simulink model "vehicleDynamicsModelTest"  (R2019b)
settings: Solver=FixedStepDiscrete  StartTime=0.0  StopTime=15  FixedStep=0.1  RelTol=1e-3
undefined symbols (not defined in the file or in its folder): DiscIntNeverNeededParam, sigbuilder_block
libraries: simulink x2
settings Model: Creator=jasprit  LastModifiedBy=jasprit
settings DataIOCC: ReturnWorkspaceOutputs=off
settings DebuggingCC: ArithmeticOperatorsInVariantConditions=warning
settings SFSimCC: CustomCodeUndefinedFunction=UseInterfaceOnly

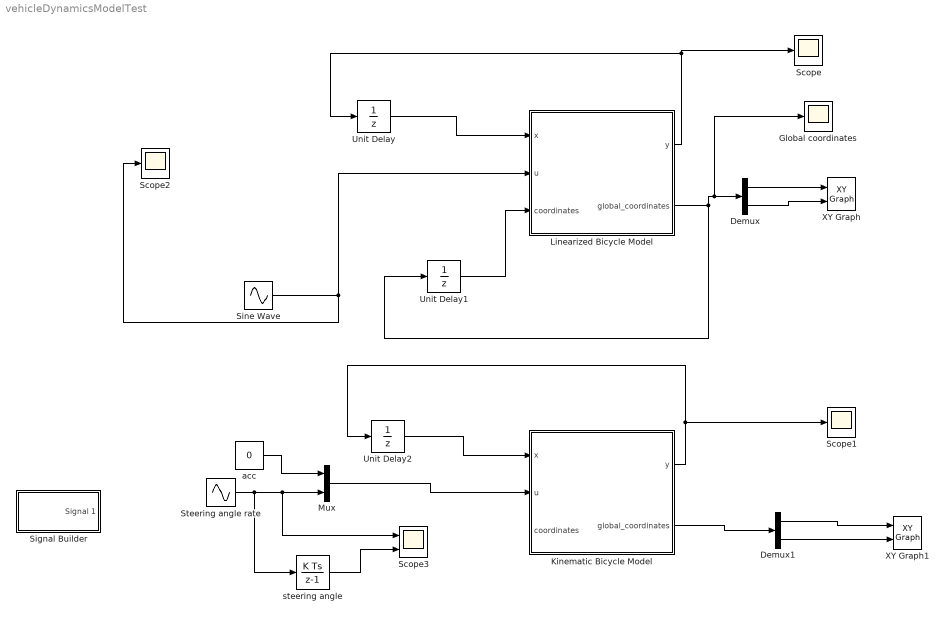
== system vehicleDynamicsModelTest ==
  Demux : Demux  Outputs=2
  Demux1 : Demux  Outputs=2
  Global coordinates : Scope
  Kinematic Bicycle Model : MATLAB Function  TreatAsAtomicUnit=on
  Linearized Bicycle Model : MATLAB Function  TreatAsAtomicUnit=on
  Mux : Mux  Inputs=2
  Scope : Scope
  Scope1 : Scope
  Scope2 : Scope
  Scope3 : Scope  NumInputPorts=2
  Signal Builder : Subsystem  Tag=STV Subsys  LoadFcn=sigbuilder_block('load');  StartFcn=sigbuilder_block('start');  StopFcn=sigbuilder_block('stop');  ClipboardFcn=sigbuilder_block('clipboard');  mask(Sigbuilder block){tuvar=[0:10]}
      mask help: Simulink:masks:SigbuilderBlock_MD
      mask init:
      | if ~strcmp(get_param(bdroot(gcbh),'SimulationStatus'),'stopped') tuvar = sigbuilder_block('maskInit'); end
      settings: CopyFcn=sigbuilder_block('copy');  DeleteFcn=sigbuilder_block('delete');  ModelCloseFcn=sigbuilder_block('modelClose');  PreSaveFcn=sigbuilder_block('preSave');  PauseFcn=sigbuilder_block('pause');  ContinueFcn=sigbuilder_block('continue');  NameChangeFcn=sigbuilder_block('namechange');  OpenFcn=sigbuilder_block('open',[414.75 52.5 588 512.25 ]);  CloseFcn=sigbuilder_block('close');
      mask Display: plot(0, 0, 100, 100,[2, 2, 32, 32, 2], [68, 8, 8, 68, 68],[32, 2], [38, 38], [32, 19, 2],[53, 60, 44], [32, 17, 17, 2],[16, 16, 31, 31]);txt = getActiveGroup(gcbh);text(2, 100, txt,'verticalAlignment', 'top');
  Sine Wave : Sin  Amplitude=0.019  Frequency=2*pi*1/10  Phase=pi/2  SampleTime=0
  Steering angle rate : Sin  Amplitude=0.0255  Frequency=2*pi/5  Phase=pi/2  SampleTime=0
  Unit Delay : UnitDelay  InitialCondition=[0; 0; 0; 0]  SampleTime=-1  HasFrameUpgradeWarning=on
  Unit Delay1 : UnitDelay  InitialCondition=[0;0]  SampleTime=-1  HasFrameUpgradeWarning=on
  Unit Delay2 : UnitDelay  InitialCondition=[0; 0; 0; 10; 0]  SampleTime=-1  HasFrameUpgradeWarning=on
  XY Graph : simulink/Sinks/XY Graph  xmin=-100  xmax=400  ymin=-10  ymax=10  st=-1
  XY Graph1 : simulink/Sinks/XY Graph  xmin=-10  xmax=200  ymin=-5  ymax=5  st=-1
  acc : Constant  Value=0
  steering angle : DiscreteIntegrator  SampleTime=-1  ICPrevOutput=DiscIntNeverNeededParam  ICPrevScaledInput=DiscIntNeverNeededParam
  wires:
  Unit Delay/1 -> Linearized Bicycle Model/1(x)
  Linearized Bicycle Model/1(y) -> Scope/1, Unit Delay/1
  Linearized Bicycle Model/2(global_coordinates) -> Unit Delay1/1, Global coordinates/1, Demux/1
  Demux/1 -> XY Graph/1
  Demux/2 -> XY Graph/2
  Unit Delay1/1 -> Linearized Bicycle Model/3(coordinates)
  Sine Wave/1 -> Linearized Bicycle Model/2(u), Scope2/1
  acc/1 -> Mux/1
  Mux/1 -> Kinematic Bicycle Model/2(u)
  Unit Delay2/1 -> Kinematic Bicycle Model/1(x)
  Kinematic Bicycle Model/1(y) -> Scope1/1, Unit Delay2/1
  Kinematic Bicycle Model/2(global_coordinates) -> Demux1/1
  Demux1/2 -> XY Graph1/2
  Demux1/1 -> XY Graph1/1
  Steering angle rate/1 -> steering angle/1, Scope3/1, Mux/2
  steering angle/1 -> Scope3/2

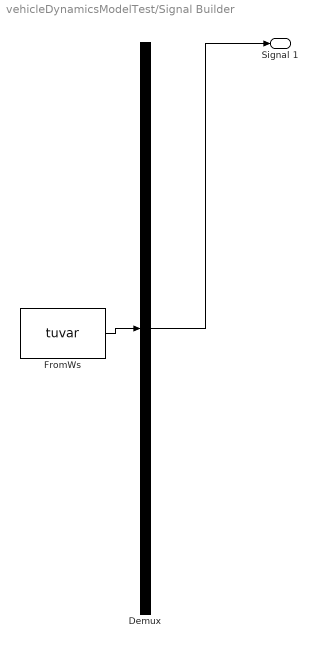
== system vehicleDynamicsModelTest/Signal Builder ==
  Demux : Demux  Tag=STV Demux  Outputs=1
  FromWs : FromWorkspace  Tag=STV FromWs  VariableName=tuvar  SampleTime=0
      SigBuilderData=|
      | common.afterFinalStr = 'Extrapolate'
      | common.sampleTime = 0
      | dataSet.timeRange = [0 10]
      | dataSet.name = 'Group 1'
      | sbobj.Groups.Name = 'Group 1'
      | sbobj.Groups.Signals.Name = 'Signal 1'
      | sbobj.Groups.Signals.XData = [0 4 4 6 6 10]
      | sbobj.Groups.Signals.YData = [0 0 0.01 0.01 0 0]
  Signal 1 : Outport  Tag=STV Outport  VectorParamsAs1DForOutWhenUnconnected=off
  wires:
  Demux/1 -> Signal 1/1
  FromWs/1 -> Demux/1

== matlab function vehicleDynamicsModelTest/Kinematic Bicycle Model ==
  data: x input; u input; y output; global_coordinates output; coordinates input
function [y, global_coordinates] = runKinematicVehicle(x, u, coordinates)
    persistent vehicleModel;
    
    Ts = .1;
    if isempty(vehicleModel)
        vehicleModel = SimplifiedKinematicBicycleModel(Ts);
    end
    
    y = vehicleModel.propagate(x, u);
    
%     vel_x = vehicleModel.V;
%     psi = y(3);
%     
%     X = vel_x * cos(psi) * Ts + coordinates(1);
%     Y = vel_x * sin(psi) * Ts + coordinates(2);
    
    global_coordinates = [y(1); y(2)];
    
end

== matlab function vehicleDynamicsModelTest/Linearized Bicycle Model ==
  data: x input; u input; y output; global_coordinates output; coordinates input
function [y, global_coordinates] = runVehicle(x, u, coordinates)
    persistent vehicleModel;
    
    Ts = .1;
    if isempty(vehicleModel)
        vehicleModel = LinearizedBicycleModel(Ts, 10);
    end
    
    y = vehicleModel.propagate(x, u);
    
    vel_x = vehicleModel.V;
    psi = y(3);
    
    X = vel_x * cos(psi) * Ts + coordinates(1);
    Y = vel_x * sin(psi) * Ts + coordinates(2);
    
    global_coordinates = [X; Y];
    
end
